simulink model "DCMotor"  (Simulink 7.7)
settings: Solver=ode45  StartTime=0.0  StopTime=10.0  MaxStep=0.001  RelTol=1e-6  AbsTol=1e-4
values from neighbouring files (symbols this model uses):
  b = 5    [DCMotorDesign.m]
  c = 12    [DCMotorDesign.m]
  J = 3    [DCMotorDesign.m]
  Kp = 1    [DCMotorDesign.m]
settings Model: Creator=pjseiler  LastModifiedBy=pjseiler

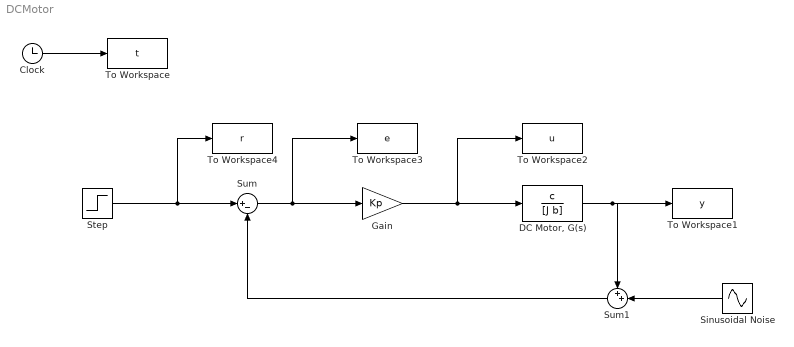
== system DCMotor ==
  Clock : Clock
      settings: Decimation=10
  "DC Motor, G(s)" : TransferFcn  Numerator=c  Denominator=[J b]
  Gain : Gain  Gain=Kp
  Sinusoidal Noise : Sin  Amplitude=0.1  Frequency=200  SampleTime=0
  Step : Step  Time=0  SampleTime=0
  Sum : Sum  Inputs=|+-
  Sum1 : Sum  Inputs=++|
  To Workspace : ToWorkspace  VariableName=t  SampleTime=-1  SaveFormat=Array
  To Workspace1 : ToWorkspace  VariableName=y  SampleTime=-1  SaveFormat=Array
  To Workspace2 : ToWorkspace  VariableName=u  SampleTime=-1  SaveFormat=Array
  To Workspace3 : ToWorkspace  VariableName=e  SampleTime=-1  SaveFormat=Array
  To Workspace4 : ToWorkspace  VariableName=r  SampleTime=-1  SaveFormat=Array
  wires:
  Sum/1 -> To Workspace3/1, Gain/1
  Clock/1 -> To Workspace/1
  "DC Motor, G(s)"/1 -> To Workspace1/1, Sum1/1
  Sum1/1 -> Sum/2
  Sinusoidal Noise/1 -> Sum1/2
  Gain/1 -> "DC Motor, G(s)"/1, To Workspace2/1
  Step/1 -> Sum/1, To Workspace4/1
